simulink model "clas_test1"  (R2015b)
settings: Solver=VariableStepAuto  StartTime=0.0  StopTime=80.0  RelTol=1e-3
values from neighbouring files (symbols this model uses):
  denc = conv(conv([0.0001 1],[0.0001 1]),[0.0001 1])    [classic_controller.m]
  gainc = 0.9    [classic_controller.m]
  Greal = sysic    [model_building.m]
  numc = conv([10 1],[0.35 0.01 1])    [classic_controller.m]
undefined symbols (not defined in the file or in its folder): pulsazione
settings Model: Creator=michele  LastModifiedBy=michele
settings DebuggingCC: AlgebraicLoopMsg=none

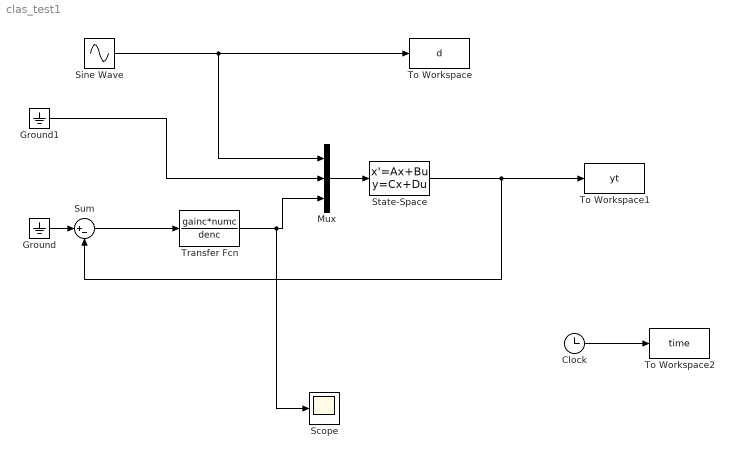
== system clas_test1 ==
  Clock : Clock
  Ground : Ground
  Ground1 : Ground
  Mux : Mux  Inputs=3
  Scope : Scope
  Sine Wave : Sin  Frequency=pulsazione  SampleTime=0
  State-Space : StateSpace  A=Greal.NominalValue.a  B=Greal.NominalValue.b  C=Greal.NominalValue.c  D=Greal.NominalValue.d  X0=0
  Sum : Sum  Inputs=|+-
  To Workspace : ToWorkspace  VariableName=d  SaveFormat=Timeseries  SampleTime=-1
  To Workspace1 : ToWorkspace  VariableName=yt  SaveFormat=Timeseries  SampleTime=-1
  To Workspace2 : ToWorkspace  VariableName=time  SaveFormat=Timeseries  SampleTime=-1
  Transfer Fcn : TransferFcn  Numerator=gainc*numc  Denominator=denc
  wires:
  Transfer Fcn/1 -> Scope/1, Mux/3
  Mux/1 -> State-Space/1
  State-Space/1 -> To Workspace1/1, Sum/2
  Sum/1 -> Transfer Fcn/1
  Ground/1 -> Sum/1
  Ground1/1 -> Mux/2
  Clock/1 -> To Workspace2/1
  Sine Wave/1 -> Mux/1, To Workspace/1
